simulink model "RLmodel"  (R2020b)
settings: Solver=VariableStepAuto  StartTime=0.0  StopTime=200  RelTol=1e-3
undefined symbols (not defined in the file or in its folder): DiscIntNeverNeededParam
libraries: rllib x1, simulink x1
settings Model: Creator=Battl  LastModifiedBy=Battl

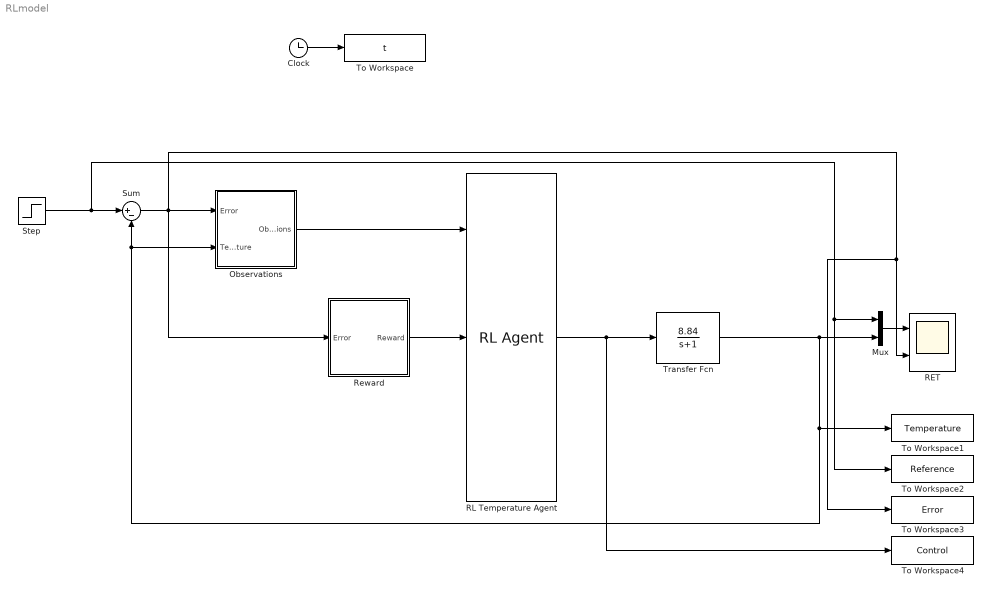
== system RLmodel ==
  Clock : Clock
  Mux : Mux  Inputs=2
  Observations : Subsystem
  RET : Scope  NumInputPorts=2
  RL Temperature Agent : rllib/RL Agent  Agent=temperature_agent  ProvideReward=on  ProvideIsDone=on  ProvideCumRwd=off  TreatAsDirectFeedthrough=on  CollectLoggedSignals=on  CollectModelStates=on
  Reward : Subsystem
  Step : Step  Time=100  Before=22.1163  After=30  SampleTime=0
  Sum : Sum  Inputs=|+-
  To Workspace : ToWorkspace  VariableName=t  SampleTime=-1
      settings: Save2DSignal=2-D array (concatenate along first dimension)
  To Workspace1 : ToWorkspace  VariableName=Temperature  SampleTime=-1
      settings: Save2DSignal=2-D array (concatenate along first dimension)
  To Workspace2 : ToWorkspace  VariableName=Reference  SampleTime=-1
      settings: Save2DSignal=2-D array (concatenate along first dimension)
  To Workspace3 : ToWorkspace  VariableName=Error  SampleTime=-1
      settings: Save2DSignal=2-D array (concatenate along first dimension)
  To Workspace4 : ToWorkspace  VariableName=Control  SampleTime=-1
      settings: Save2DSignal=2-D array (concatenate along first dimension)
  Transfer Fcn : TransferFcn  Numerator=[8.84]  Denominator=[1 1]
  wires:
  Step/1 -> To Workspace2/1, Mux/1, Sum/1
  Transfer Fcn/1 -> To Workspace1/1, Observations/2(Temperature), Sum/2, Mux/2
  Observations/1(Observations) -> RL Temperature Agent/1
  Reward/1(Reward) -> RL Temperature Agent/2
  RL Temperature Agent/1 -> To Workspace4/1, Transfer Fcn/1
  Mux/1 -> RET/1
  Clock/1 -> To Workspace/1
  Sum/1 -> To Workspace3/1, RET/2, Observations/1(Error), Reward/1(Error)

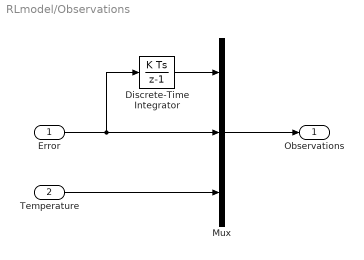
== system RLmodel/Observations ==
  Error : Inport
  Temperature : Inport  Port=2
  Discrete-Time Integrator : DiscreteIntegrator  SampleTime=-1  ICPrevOutput=DiscIntNeverNeededParam  ICPrevScaledInput=DiscIntNeverNeededParam
  Mux : Mux  Inputs=3
  Observations : Outport
  wires:
  Mux/1 -> Observations/1
  Temperature/1 -> Mux/3
  Error/1 -> Discrete-Time Integrator/1, Mux/2
  Discrete-Time Integrator/1 -> Mux/1

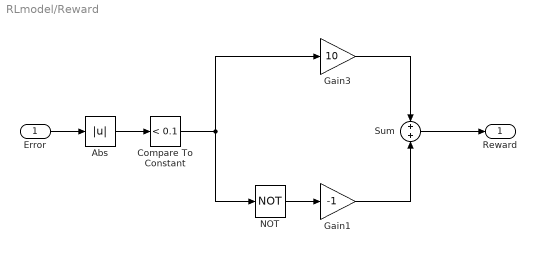
== system RLmodel/Reward ==
  Error : Inport
  Abs : Abs
  Compare To Constant : simulink/Logic and Bit Operations/Compare To Constant  relop=<  const=0.1  OutDataTypeStr=boolean
  Gain1 : Gain  Gain=-1
  Gain3 : Gain  Gain=10
  NOT : Logic  Operator=NOT  IconShape=distinctive  AllPortsSameDT=off  OutDataTypeStr=boolean
  Sum : Sum
  Reward : Outport
  wires:
  Error/1 -> Abs/1
  Abs/1 -> Compare To Constant/1
  Compare To Constant/1 -> Gain3/1, NOT/1
  NOT/1 -> Gain1/1
  Gain1/1 -> Sum/2
  Gain3/1 -> Sum/1
  Sum/1 -> Reward/1
